simulink model "Exemplu_figura8"  (R2016a)
settings: Solver=VariableStepDiscrete  StartTime=0.0  StopTime=2400  RelTol=1e-3
undefined symbols (not defined in the file): m, n
settings Model: Creator=Cristina  LastModifiedBy=Cristina

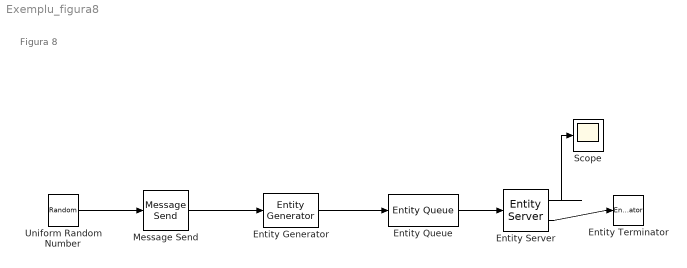
== system Exemplu_figura8 ==
  note: Figura 8
  Entity Generator : EntityGenerator  InputPortMessageModes=m  OutputPortMessageModes=m  GenerationMethod=Event-based  GenerateAction=|  AttributeName=Attribute|ServiceTime  AttributeInitialValue=1|1  EntityType=Structured  EntityTypeName=Entity
      | persistent init
      | if (isempty(init))
      |     rng(2347);
      |     init = true;
      | end
      | entity.ServiceTime = 3.5 + rand * 3;
      settings: InputPortMap=u0
  Entity Queue : EntityQueue  InputPortMessageModes=m  OutputPortMessageModes=m
      settings: OutputPortMap=o5
  Entity Server : EntityServer  InputPortMessageModes=m  OutputPortMessageModes=n,m  Capacity=1  ServiceTimeSource=Attribute  AverageWait=on
      settings: OutputPortMap=o4,o9
  Entity Terminator : EntityTerminator  InputPortMessageModes=m
  Message Send : MessageSend  OutputPortMessageModes=m
      settings: InputPortMap=u1
  Scope : Scope
  Uniform Random Number : UniformRandomNumber  SampleTime=0.1
  wires:
  Uniform Random Number/1 -> Message Send/1
  Message Send/1 -> Entity Generator/1
  Entity Generator/1 -> Entity Queue/1
  Entity Queue/1 -> Entity Server/1
  Entity Server/2 -> Entity Terminator/1
  Entity Server/1 -> Scope/1
